simulink model "VCU_CS75_12_16_Test"  (R2014a)
settings: Solver=FixedStepDiscrete  StartTime=0.0  StopTime=25  FixedStep=0.0005  RelTol=1e-3
undefined symbols (not defined in the file): ecucoder_acal, I_SW01_L, LaterlAngleCommand, LDW, RemoteAcclPosition
libraries: simulink x913, ec5744lib x39
(part 1 of 30)
settings Model: Creator=pc  LastModifiedBy=ZJK
settings OptimizationCC: InlineParams=on  InlineInvariantSignals=on  ExpressionFolding=off  RollThreshold=9  StateBitsets=on  DataBitsets=on  UseTempVars=on  ZeroExternalMemoryAtStartup=off  ZeroInternalMemoryAtStartup=off  EfficientFloat2IntCast=on  OptimizeModelRefInitCode=on  LifeSpan=1
settings DebuggingCC: InheritedTsInSrcMsg=none  MultiTaskDSMMsg=none
settings HardwareCC: ProdLargestAtomicInteger=Long  ProdLargestAtomicFloat=Double  ProdIntDivRoundTo=Zero  ProdEndianess=BigEndian  ProdHWDeviceType=Freescale MPC5500
settings RTWCC: SystemTargetFile=ec5744.tlc  MakeCommand=make_rtw optimized_fixed_point=1  GenerateMakefile=off  TemplateMakefile=ec5744_lcc.tmf  PostCodeGenCommand=ec5744_pst_s2(buildInfo)  Description=Target for EC5744  GenerateReport=on  ProcessScript=ec5744_make_rtw_hook  IncludeHyperlinkInReport=on  LaunchReport=on
settings CodeAppCC: IgnoreCustomStorageClasses=off
settings STFCustomTargetCC: ModelReferenceCompliant=off  ConcurrentExecutionCompliant=off  IncludeMdlTerminateFcn=off  GeneratePreprocessorConditionals=Use local settings  CombineOutputUpdateFcns=on  SuppressErrorStatus=on  ERTCustomFileBanners=on  SupportContinuousTime=off  SupportNonInlinedSFcns=off  MATLABClassNameForMDSCustomization=Simulink.SoftwareTarget.ERTCustomization  GRTInterface=off  SystemTargetFile=ec5744.tlc
settings ERTTargetCC: GenerateSampleERTMain=off  ModelReferenceCompliant=off  IncludeMdlTerminateFcn=off  SuppressErrorStatus=on  GenerateASAP2=on  ERTSrcFileBannerTemplate=ec5744_code_template.cgt  ERTHdrFileBannerTemplate=ec5744_code_template.cgt  ERTDataSrcFileTemplate=ec5744_code_template.cgt  ERTDataHdrFileTemplate=ec5744_code_template.cgt  ERTCustomFileTemplate=ec5744_file_process.tlc

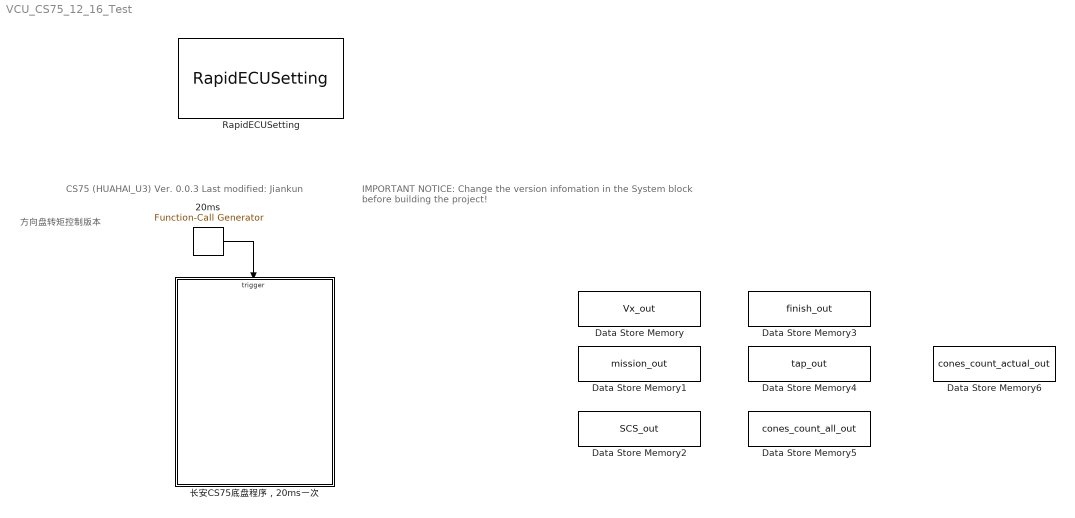
== system VCU_CS75_12_16_Test ==
  note: 方向盘转矩控制版本
  note: CS75 (HUAHAI_U3)
      | Ver. 0.0.3
      | Last modified: Jiankun
  note: IMPORTANT NOTICE:
      | Change the version infomation in the System block
      | before building the project!
  20ms : simulink/Ports & Subsystems/Function-Call Generator  sample_time=0.02  numberOfIterations=1
  Data Store Memory : DataStoreMemory  DataStoreName=Vx_out  ReadBeforeWriteMsg=warning  WriteAfterWriteMsg=warning  WriteAfterReadMsg=warning
  Data Store Memory1 : DataStoreMemory  DataStoreName=mission_out  ReadBeforeWriteMsg=warning  WriteAfterWriteMsg=warning  WriteAfterReadMsg=warning
  Data Store Memory2 : DataStoreMemory  DataStoreName=SCS_out  ReadBeforeWriteMsg=warning  WriteAfterWriteMsg=warning  WriteAfterReadMsg=warning
  Data Store Memory3 : DataStoreMemory  DataStoreName=finish_out  ReadBeforeWriteMsg=warning  WriteAfterWriteMsg=warning  WriteAfterReadMsg=warning
  Data Store Memory4 : DataStoreMemory  DataStoreName=tap_out  ReadBeforeWriteMsg=warning  WriteAfterWriteMsg=warning  WriteAfterReadMsg=warning
  Data Store Memory5 : DataStoreMemory  DataStoreName=cones_count_all_out  ReadBeforeWriteMsg=warning  WriteAfterWriteMsg=warning  WriteAfterReadMsg=warning
  Data Store Memory6 : DataStoreMemory  DataStoreName=cones_count_actual_out  ReadBeforeWriteMsg=warning  WriteAfterWriteMsg=warning  WriteAfterReadMsg=warning
  RapidECUSetting : ec5744lib/RapidECU_U3/RapidECUSetting
      link override CAN: apdf=4  bpdf=4  cpdf=4  acmt=Extended(29-bit ID)
      link override LIN: abrt=19200
  长安CS75底盘程序，20ms一次 : Subsystem
  wires:
  20ms/1 -> 长安CS75底盘程序，20ms一次/Trigger

== system VCU_CS75_12_16_Test/长安CS75底盘程序，20ms一次 ==
  Trigger : TriggerPort  TriggerType=function-call  PortDimensions=1
  APP : Subsystem  TreatAsAtomicUnit=on
  Input : Subsystem  TreatAsAtomicUnit=on
  Output : Subsystem
  wires:
  Input/1(IO_Input) -> APP/1(APP_Input)
  APP/1(APP_Output) -> Output/1(IO_Output)

== system VCU_CS75_12_16_Test/长安CS75底盘程序，20ms一次/APP ==
  note: 完全调试完需要修改一下，目前这个模块无用
  note: APP Module
      | Ver. 0.0.2
      | Last modified: ZJK 2020-10-09
  APP_Input : Inport
  Bus Creator1 : BusCreator
  Controller : Subsystem
  Monitor : Subsystem
  System_State_Manager : Subsystem
  APP_Output : Outport
  wires:
  Bus Creator1/1 -> APP_Output/1
  System_State_Manager/1(System_State) -> Bus Creator1/2, Controller/3(System_State)  "System_State"
  Monitor/1(System_Status) -> Bus Creator1/3, System_State_Manager/1(System_Status), Controller/2(System_Status)  "System_Status"
  Controller/1(Control_Output) -> Bus Creator1/1  "Control_Output"
  APP_Input/1 -> Controller/1(APP_Input), Bus Creator1/4, Monitor/1(APP_Input)  "APP_Input"

== system VCU_CS75_12_16_Test/长安CS75底盘程序，20ms一次/Input ==
  note: 程序版本-------方向盘转矩控制版本
  note: 接收底层发来的Messages
  note: 接收服务器Messages
  note: 低有效开关量6，用作横向自动驾驶开关
  note: Module
      | Ver. 0.0.1
      | Last modified by ZJK
  ADC_Input : Subsystem
  Bus Creator : BusCreator
  CAN0_Rx : Subsystem
  CAN1_Rx : Subsystem
  DBC转化的messages（存底） : Subsystem  Commented=on
  System : Subsystem  TreatAsAtomicUnit=on
  IO_Input : Outport
  wires:
  CAN0_Rx/1(CAN0_Data_Rx) -> Bus Creator/1  "CAN0_Data_Rx"
  CAN1_Rx/1(CAN1_Data_Rx) -> Bus Creator/2  "CAN1_Data_Rx"
  System/1(System_Output) -> Bus Creator/3  "System_Output"
  ADC_Input/1(ADC_Input) -> Bus Creator/4  "ADC_Input"
  Bus Creator/1 -> IO_Input/1

== system VCU_CS75_12_16_Test/长安CS75底盘程序，20ms一次/Output ==
  IO_Output : Inport
  CAN0_Tx : Subsystem
  CAN1_Tx : Subsystem
  Subsystem : Subsystem  Commented=on
  wires:
  IO_Output/1 -> CAN0_Tx/1(APP_Out), CAN1_Tx/1(APP_Out)

== system VCU_CS75_12_16_Test/长安CS75底盘程序，20ms一次/APP/Controller ==
  note: 方向盘震动控制，在退出和进入自动驾驶启用，目前未启用
  APP_Input : Inport
  System_Status : Inport  Port=2
  System_State : Inport  Port=3
  Accesories : Subsystem  TreatAsAtomicUnit=on
  Bus Creator : BusCreator  Inputs=5
  Bus Creator2 : BusCreator
  Bus Selector : BusSelector  OutputSignals=CAN0_Data_Rx,CAN1_Data_Rx,ADC_Input
  General : Subsystem  Commented=on  TreatAsAtomicUnit=on
  Lateral : Subsystem  TreatAsAtomicUnit=on
  Longitudinal : Subsystem  TreatAsAtomicUnit=on
  Control_Output : Outport
  wires:
  Bus Creator/1 -> General/1(Control_Input), Longitudinal/1(Control_Input), Accesories/1(Control_Input), Lateral/1(Control_Input)  "Control_Input"
  Bus Selector/1 -> Bus Creator/1  "<CAN0_Data_Rx>"
  APP_Input/1 -> Bus Selector/1
  Bus Selector/2 -> Bus Creator/2  "<CAN1_Data_Rx>"
  Accesories/1(Accesories_Output) -> Bus Creator2/4  "Accesories_Output"
  Lateral/1(Lateral_Output) -> Bus Creator2/3  "Lateral_Output"
  General/1(General_Output) -> Bus Creator2/1  "General_Output"
  Longitudinal/1(Longitudinal_Output) -> Bus Creator2/2  "Longitudinal_Output"
  Bus Creator2/1 -> Control_Output/1  "Control_Output"
  System_Status/1 -> Bus Creator/4  "System_Status"
  Bus Selector/3 -> Bus Creator/3  "<ADC_Input>"
  System_State/1 -> Bus Creator/5  "System_State"

== system VCU_CS75_12_16_Test/长安CS75底盘程序，20ms一次/APP/Monitor ==
  note: 网关发出EPS\ESP通讯或功能故障
  note: 人工接管状态（只要是制动踏板踩下，就认为驾驶员在控车）
  note: 服务器的通信状态/服务器下发的Ready信号
  note: 底层自己装的一个Switch，低有效
      | 可能用于判定进入自动驾驶的一个信号
  APP_Input : Inport
  Bus Creator : BusCreator
  Server_Status : Subsystem
  Switches_Status : Subsystem
  Vehicle_Status : Subsystem
  Vehicle_Takeover_Status : Subsystem
  System_Status : Outport
  wires:
  Bus Creator/1 -> System_Status/1
  APP_Input/1 -> [APP_Input]
  [APP_Input] -> Vehicle_Status/1(APP_Input)
  [APP_Input] -> Switches_Status/1(APP_Input)
  [APP_Input] -> Server_Status/1(APP_Input)
  [APP_Input] -> Vehicle_Takeover_Status/1(APP_Input)
  Vehicle_Status/1(Vehicle_Status) -> Bus Creator/1  "VehicleStatus"
  Vehicle_Takeover_Status/1(Takeover_Status) -> Bus Creator/2  "TakeOver1"
  Server_Status/1(Server_Status) -> Bus Creator/3  "ServerStatus"
  Switches_Status/1(Switches_Status) -> Bus Creator/4  "Switch_Status"

== system VCU_CS75_12_16_Test/长安CS75底盘程序，20ms一次/APP/System_State_Manager ==
  note: 暂时不考虑横向自动驾驶，目的是调试横向PID
  note: 0：人工驾驶；
      | 1：纵向自动驾驶；
      | 2：人工接管；
      | 3：底盘通信故障/功能故障；需要人工接管；
  System_Status : Inport
  Bus Selector : BusSelector  OutputSignals=VehicleStatus.VehicleFaultStatus,VehicleStatus.VehicleCommunicationStatus,VehicleStatus.EPS_AvailabilityStatus,TakeOver1,ServerStatus.Server_CommunicationStatus,ServerStatus.AutoDrivingReady,Switch_Status.P6_Value
  Chart : Stateflow chart  TreatAsAtomicUnit=on
  System_State : Outport
  wires:
  System_Status/1 -> Bus Selector/1
  Bus Selector/1 -> Chart/1(VehicleFaultStatus)  "<VehicleFaultStatus>"
  Bus Selector/2 -> Chart/2(VehicleComminicationStatus)  "<VehicleCommunicationStatus>"
  Bus Selector/4 -> Chart/4(TakeoverStatus)  "<TakeOver1>"
  Bus Selector/5 -> Chart/5(Server_CommunicationStatus)  "<Server_CommunicationStatus>"
  Bus Selector/6 -> Chart/6(AutoDrivingReady)  "<AutoDrivingReady>"
  Chart/1(System_State) -> System_State/1  "System_State"
  Bus Selector/7 -> Chart/7(Switch_P6)  "<P6_Value>"
  Bus Selector/3 -> Chart/3(EPS_AvailabilityStatus)  "<EPS_AvailabilityStatus>"

== system VCU_CS75_12_16_Test/长安CS75底盘程序，20ms一次/Input/ADC_Input ==
  Bus Creator2 : BusCreator  Inputs=1
  Data Type Conversion : DataTypeConversion  OutDataTypeStr=double
  MATLAB Function : MATLAB Function  TreatAsAtomicUnit=on
  SwitchInput : ec5744lib/RapidECU_U3/01BasicInput/SwitchInput  channel=6:I_SW01_L  sampletime=-1
  ADC_Input : Outport
  wires:
  SwitchInput/1 -> Data Type Conversion/1  "P6_Value"
  Bus Creator2/1 -> ADC_Input/1  "ADC_Input"
  Data Type Conversion/1 -> MATLAB Function/1(u)  "P6_Value"
  MATLAB Function/1(y) -> Bus Creator2/1  "P6_Value"

== system VCU_CS75_12_16_Test/长安CS75底盘程序，20ms一次/Input/CAN0_Rx ==
  note: BSW CAN 1 Receive
      | Communication to the vehicle
      | Ver. 1.0
      | 2020/11/14
  Bus Creator : BusCreator  Commented=on  Inputs=5
  Bus Creator2 : BusCreator  Inputs=1
  Constant : Constant  Commented=on  Value=0  SampleTime=-1
  Constant1 : Constant  Commented=on  Value=0  SampleTime=-1
  Constant2 : Constant  Commented=on  Value=0  SampleTime=-1
  ECCalVar1 : Constant  Commented=on  InitFcn=ecucoder_acal;  Value=RemoteAcclPosition  OutDataTypeStr=Inherit: Inherit via back propagation  SampleTime=-1
  ECCalVar2 : Constant  Commented=on  InitFcn=ecucoder_acal;  Value=LaterlAngleCommand  OutDataTypeStr=Inherit: Inherit via back propagation  SampleTime=-1
  a1_211 : Subsystem
  CAN0_Data_Rx : Outport
  wires:
  [A1_211] -> Bus Creator2/1  "A1_Data"
  Bus Creator2/1 -> CAN0_Data_Rx/1  "CAN0_Data_Rx"
  Bus Creator/1 -> ?
  Constant2/1 -> Bus Creator/1  "AutoDrivingReady"
  ECCalVar1/1 -> Bus Creator/2  "RemoteAcclPosition"
  ECCalVar2/1 -> Bus Creator/3  "LaterlAngleCommand"
  Constant/1 -> Bus Creator/4  "A1_Message_Counter"
  Constant1/1 -> Bus Creator/5  "A1_Checksum"
  a1_211/1(A1_211) -> [A1_211]

== system VCU_CS75_12_16_Test/长安CS75底盘程序，20ms一次/Input/CAN1_Rx ==
  BCM_288 : Subsystem
  BCM_328 : Subsystem
  BCM_348 : Subsystem
  BCM_3DF : Subsystem
  Bus Creator2 : BusCreator  Inputs=27
  EMS_205 : Subsystem
  EMS_255 : Subsystem
  EMS_265 : Subsystem
  EMS_276 : Subsystem
  EPB_256 : Subsystem
  EPS_20A : Subsystem
  EPS_21A : Subsystem
  ESP_277 : Subsystem
  ESP_280 : Subsystem
  ESP_281 : Subsystem
  ESP_287 : Subsystem
  GW_20B : Subsystem
  GW_308 : Subsystem
  GW_332 : Subsystem
  GW_376 : Subsystem
  GW_3A2 : Subsystem
  GW_567 : Subsystem
  HU_GPS_500 : Subsystem
  LAS_36E : Subsystem
  SAS_108 : Subsystem
  SCM_3B8 : Subsystem
  SRS_005 : Subsystem
  TCU_286 : Subsystem
  CAN1_Data_Rx : Outport
  wires:
  Bus Creator2/1 -> CAN1_Data_Rx/1  "CAN1_Data_Rx"
  [SAS_108] -> Bus Creator2/11  "SAS_108_Data"
  [BCM_328] -> Bus Creator2/16  "BCM_328_Data"
  [SCM_3B8] -> Bus Creator2/12  "SCM_3B8_Data"
  [GW_308] -> Bus Creator2/21  "GW_308_Data"
  [EMS_265] -> Bus Creator2/3  "EMS_265_Data"
  [ESP_287] -> Bus Creator2/10  "ESP_287_Data"
  [EPS_21A] -> Bus Creator2/6  "EPS_21A_Data"
  [ESP_277] -> Bus Creator2/7  "ESP_277_Data"
  [BCM_3DF] -> Bus Creator2/18  "BCM_3DF_Data"
  [ESP_281] -> Bus Creator2/9  "ESP_281_Data"
  [GW_332] -> Bus Creator2/20  "GW_332_Data"
  [ESP_280] -> Bus Creator2/8  "ESP_280_Data"
  [GW_20B] -> Bus Creator2/19  "GW_20B_Data"
  [BCM_348] -> Bus Creator2/17  "BCM_348_Data"
  [GW_376] -> Bus Creator2/22  "GW_376_Data"
  [SRS_005] -> Bus Creator2/13  "SRS_005_Data"
  [BCM_288] -> Bus Creator2/15  "BCM_288_Data"
  [TCU_286] -> Bus Creator2/14  "TCU_286_Data"
  [EPS_20A] -> Bus Creator2/5  "EPS_20A_Data"
  [EPB_256] -> Bus Creator2/4  "EPB_256_Data"
  [GW_3A2] -> Bus Creator2/23  "GW_3A2_Data"
  [GW_567] -> Bus Creator2/24  "GW_567_Data"
  [HU_GPS_500] -> Bus Creator2/25  "HU_GPS_500_Data"
  [LAS_36E] -> Bus Creator2/26  "LAS_36E_Data"
  [EMS_276] -> Bus Creator2/27  "EMS_276_Data"
  [EMS_205] -> Bus Creator2/1  "EMS_205_Data"
  [EMS_255] -> Bus Creator2/2  "EMS_255_Data"
  EMS_255/1(EMS_255) -> [EMS_255]
  EMS_265/1(EMS_265) -> [EMS_265]
  EMS_276/1(EMS_276) -> [EMS_276]
  EPB_256/1(EPB_256) -> [EPB_256]
  EMS_205/1(EMS_205) -> [EMS_205]
  EPS_20A/1(EPS_20A) -> [EPS_20A]
  EPS_21A/1(EPS_21A) -> [EPS_21A]
  ESP_277/1(ESP_277) -> [ESP_277]
  ESP_280/1(ESP_280) -> [ESP_280]
  ESP_281/1(ESP_281) -> [ESP_281]
  ESP_287/1(ESP_287) -> [ESP_287]
  SAS_108/1(SAS_108) -> [SAS_108]
  SCM_3B8/1(SCM_3B8) -> [SCM_3B8]
  SRS_005/1(SRS_005) -> [SRS_005]
  TCU_286/1(TCU_286) -> [TCU_286]
  BCM_288/1(BCM_288) -> [BCM_288]
  BCM_328/1(BCM_328) -> [BCM_328]
  BCM_348/1(BCM_348) -> [BCM_348]
  BCM_3DF/1(BCM_3DF) -> [BCM_3DF]
  GW_20B/1(GW_20B) -> [GW_20B]
  GW_332/1(GW_332) -> [GW_332]
  GW_308/1(GW_308) -> [GW_308]
  GW_376/1(GW_376) -> [GW_376]
  GW_3A2/1(GW_3A2) -> [GW_3A2]
  GW_567/1(GW_567) -> [GW_567]
  HU_GPS_500/1(HU_GPS_500) -> [HU_GPS_500]
  LAS_36E/1(LAS_36E) -> [LAS_36E]

== system VCU_CS75_12_16_Test/长安CS75底盘程序，20ms一次/Input/DBC转化的messages（存底） ==
  ReceiveMessages : Subsystem
  ReceiveMessages1 : Subsystem
  ReceiveMessages10 : Subsystem
  ReceiveMessages11 : Subsystem
  ReceiveMessages12 : Subsystem
  ReceiveMessages13 : Subsystem
  ReceiveMessages14 : Subsystem
  ReceiveMessages15 : Subsystem
  ReceiveMessages16 : Subsystem
  ReceiveMessages17 : Subsystem
  ReceiveMessages18 : Subsystem
  ReceiveMessages19 : Subsystem
  ReceiveMessages2 : Subsystem
  ReceiveMessages20 : Subsystem
  ReceiveMessages21 : Subsystem
  ReceiveMessages22 : Subsystem
  ReceiveMessages23 : Subsystem
  ReceiveMessages24 : Subsystem
  ReceiveMessages25 : Subsystem
  ReceiveMessages26 : Subsystem
  ReceiveMessages27 : Subsystem
  ReceiveMessages28 : Subsystem
  ReceiveMessages3 : Subsystem
  ReceiveMessages4 : Subsystem
  ReceiveMessages5 : Subsystem
  ReceiveMessages6 : Subsystem
  ReceiveMessages7 : Subsystem
  ReceiveMessages8 : Subsystem
  ReceiveMessages9 : Subsystem

== system VCU_CS75_12_16_Test/长安CS75底盘程序，20ms一次/Input/System ==
  Bus Creator : BusCreator  Inputs=1
  Bus Creator1 : BusCreator  Inputs=3
  Version_Major : Constant  Value=0  SampleTime=-1  LockScale=on
  Version_Minor : Constant  Value=0  SampleTime=-1
  Version_Patch : Constant  Value=2  SampleTime=-1
  System_Output : Outport
  wires:
  Bus Creator/1 -> System_Output/1  "System"
  Version_Minor/1 -> Bus Creator1/2  "Version_Minor"
  Version_Major/1 -> Bus Creator1/1  "Version_Major"
  Bus Creator1/1 -> Bus Creator/1  "Version"
  Version_Patch/1 -> Bus Creator1/3  "Version_Patch"

== system VCU_CS75_12_16_Test/长安CS75底盘程序，20ms一次/Output/CAN0_Tx ==
  note: BSW CAN0 Transmit
      | Communication to the Computer
      | Ver. 1.0
      | Last modified: ZJK 2020-10-05
  APP_Out : Inport
  From{,1..3} (4 alike) : From  Commented=on  GotoTag=APP_Signals
  to511 : Subsystem
  to6001 : Subsystem  Commented=on
  to6002 : Subsystem  Commented=on
  to6003 : Subsystem  Commented=on
  to6004 : Subsystem  Commented=on
  to601 : Subsystem
  wires:
  From/1 -> to6001/1(APP_Signals)
  APP_Out/1 -> [APP_Signals]
  From1/1 -> to6002/1(APP_Signals)
  From2/1 -> to6003/1(APP_Signals)
  From3/1 -> to6004/1(APP_Signals)
  [APP_Signals] -> to511/1(APP_Signals)
  [APP_Signals] -> to601/1(APP_Signals)

== system VCU_CS75_12_16_Test/长安CS75底盘程序，20ms一次/Output/CAN1_Tx ==
  note: BSW CAN 1 Transmit
      | Communication to the vehicle
      | Ver. 1.0
      | Last modified: ZJK 2020-
  APP_Out : Inport
  Bus Selector : BusSelector  Commented=on  OutputSignals=System_Status.Switch_Status.P6_Value
  From4 : From  Commented=on  GotoTag=APP_Signals
  Switch Case : SwitchCase  Commented=on  CaseConditions={0,1}  ShowDefaultCase=off
  Terminator : Terminator  Commented=on
  to28D : Subsystem
  to2E4 : Subsystem
  to2E5 : Subsystem
  wires:
  APP_Out/1 -> [APP_Signals]
  [APP_Signals] -> to2E4/1(APP_Signals)
  [APP_Signals] -> to2E5/1(APP_Signals)
  Switch Case/2 -> ?
  [APP_Signals] -> to28D/1(APP_Signals)
  From4/1 -> Bus Selector/1
  Bus Selector/1 -> Switch Case/1  "<P6_Value>"
  Switch Case/1 -> Terminator/1

== system VCU_CS75_12_16_Test/长安CS75底盘程序，20ms一次/Output/Subsystem ==
  28A : Subsystem
  28D : Subsystem
  2E4 : Subsystem
  2E5 : Subsystem
  TransmitMessages1 : Subsystem
  TransmitMessages10 : Subsystem
  TransmitMessages11 : Subsystem
  TransmitMessages13 : Subsystem
  TransmitMessages14 : Subsystem
  TransmitMessages2 : Subsystem
  TransmitMessages3 : Subsystem
  TransmitMessages4 : Subsystem
  TransmitMessages5 : Subsystem
  TransmitMessages7 : Subsystem
  TransmitMessages8 : Subsystem

== system VCU_CS75_12_16_Test/长安CS75底盘程序，20ms一次/APP/Controller/Accesories ==
  note: ID:28D
  note: 这里只有一个附加功能，方向盘震动；
      | 自己可以添加其他功能
  Control_Input : Inport
  Bus Creator : BusCreator  Inputs=2
  Bus Selector : BusSelector  OutputSignals=System_State
  ECCalVar : Constant  InitFcn=ecucoder_acal;  Value=LDW  OutDataTypeStr=Inherit: Inherit via back propagation  SampleTime=-1
  MATLAB Function : MATLAB Function  TreatAsAtomicUnit=on
  MATLAB Function1 : MATLAB Function  TreatAsAtomicUnit=on
  MATLAB Function2 : MATLAB Function  TreatAsAtomicUnit=on
  Memory2 : Memory  InheritSampleTime=on
  Accesories_Output : Outport
  wires:
  Control_Input/1 -> Bus Selector/1
  Bus Creator/1 -> Accesories_Output/1
  MATLAB Function/1(y1) -> Bus Creator/1  "LAS_LDWVibrationWarning"
  MATLAB Function/2(y2) -> Bus Creator/2  "LAS_LDWStatus"
  Memory2/1 -> MATLAB Function1/2(u2)
  Bus Selector/1 -> MATLAB Function2/1(u)  "<System_State>"
  MATLAB Function2/1(y) -> MATLAB Function1/1(u1), Memory2/1
  ECCalVar/1 -> MATLAB Function/1(u)

== system VCU_CS75_12_16_Test/长安CS75底盘程序，20ms一次/APP/Controller/General ==
  Control_Input : Inport
  Bus Creator : BusCreator  Inputs=1
  Bus Selector : BusSelector  OutputSignals=System_State
  MATLAB Function : MATLAB Function  TreatAsAtomicUnit=on
  General_Output : Outport
  wires:
  Bus Creator/1 -> General_Output/1
  MATLAB Function/1(y) -> Bus Creator/1  "ControlMode"
  Bus Selector/1 -> MATLAB Function/1(u)  "<System_State>"
  Control_Input/1 -> Bus Selector/1

== system VCU_CS75_12_16_Test/长安CS75底盘程序，20ms一次/APP/Controller/Lateral ==
  note: 查表
  note: 方向盘转角
  note: 轮胎转角
  note: 进入PID的信号
  note: 转矩输出
  note: 方向盘实际转角
  note: 目标控制转角
  note: 积分限幅
  note: 反馈的方向盘转角
  note: 转矩限幅
  note: 横向自动驾驶开关
  note: 转矩控制转向
  note: 位置式PID output = P*Error + I*ErrorSum + D*(Error - ErrorPre)
  note: 斜率控制，这里20才能让EPS不报警
  Control_Input : Inport
  1-D Lookup Table : Lookup_n-D  NumberOfTableDimensions=1  BreakpointsForDimension1=[-100 100]  Table=[-500 500]  InternalRulePriority=Speed  RndMeth=Simplest  InputSameDT=on
  Bus Creator1 : BusCreator  Inputs=6
  Bus Selector : BusSelector  OutputSignals=System_State,CAN0_Data_Rx.A1_Data.LaterlAngleCommand,System_Status.Switch_Status.P6_Value,CAN1_Data_Rx.TCU_286_Data.TCU_ActualGear,CAN1_Data_Rx.SAS_108_Data.SAS_SteeringAngle
  Constant : Constant  Value=0  SampleTime=-1
  Constant1 : Constant  SampleTime=-1
  Constant2 : Constant  Value=4  SampleTime=-1
  Constant3 : Constant  Value=0.2  SampleTime=-1
  Constant4 : Constant  Value=0  SampleTime=-1
  Constant5 : Constant  Value=1500  SampleTime=-1
  Constant6 : Constant  Value=3  SampleTime=-1
  Constant7 : Constant  Value=20  SampleTime=-1
  Data Type Conversion{1..4} (4 alike) : DataTypeConversion
  Gain1 : Gain  Gain=0.01
  MATLAB Function : MATLAB Function  TreatAsAtomicUnit=on
  MATLAB Function1 : MATLAB Function  TreatAsAtomicUnit=on
  MATLAB Function2 : MATLAB Function  TreatAsAtomicUnit=on
  MATLAB Function3 : MATLAB Function  TreatAsAtomicUnit=on
  MATLAB Function4 : MATLAB Function  TreatAsAtomicUnit=on
  MATLAB Function7 : MATLAB Function  TreatAsAtomicUnit=on
  Memory{1..4} (4 alike) : Memory  InheritSampleTime=on
  Switch : Switch  Criteria=u2 > Threshold
  Terminator : Terminator
  Lateral_Output : Outport
  wires:
  Control_Input/1 -> Bus Selector/1
  Bus Creator1/1 -> Lateral_Output/1  "28D"
  Bus Selector/2 -> [LaterlTorqueCommand]  "<LaterlAngleCommand>"
  Memory2/1 -> MATLAB Function2/2(LastCounter)
  Bus Selector/1 -> [System_State], MATLAB Function7/1(u)  "<System_State>"
  MATLAB Function7/1(y) -> [AutoDrivingMode]
  Bus Selector/3 -> [P6_Vaule]  "<P6_Value>"
  MATLAB Function3/1(LAS_Status) -> Bus Creator1/2  "LAS_LKSStatus"
  Bus Selector/4 -> [TCU_ActualGear]  "<TCU_ActualGear>"
  MATLAB Function4/1(y) -> Bus Creator1/1  "LAS_SteeringTorque"
  [System_State] -> MATLAB Function3/2(System_State)
  [P6_Vaule] -> MATLAB Function3/1(P6)
  Bus Selector/5 -> [SAS_SteeringAngle]  "<SAS_SteeringAngle>"
  [P6_Vaule] -> Switch/2
  Constant/1 -> Switch/3
  Switch/1 -> MATLAB Function4/1(T)
  Constant1/1 -> MATLAB Function2/1(Ready)
  MATLAB Function3/2(LateralTakeover) -> Terminator/1
  MATLAB Function2/1(RollingCounter) -> Memory2/1, Bus Creator1/3  "LAS_RollingCounter"
  [LaterlTorqueCommand] -> 1-D Lookup Table/1
  [SAS_SteeringAngle] -> MATLAB Function/2(SAS_SteeringAngle)
  [P6_Vaule] -> MATLAB Function/3(Ready)
  MATLAB Function/1(SteeringTorqueOut) -> MATLAB Function1/2(u1)  "PID_SteeringOut"
  MATLAB Function/3(ErrorSum) -> Data Type Conversion1/1  "ErrorSum"
  MATLAB Function/2(Error) -> Data Type Conversion2/1  "Error"
  Constant4/1 -> MATLAB Function/6(D)
  1-D Lookup Table/1 -> MATLAB Function/1(LaterlAngleCommand)  "mubiao_zhuanjiao"
  MATLAB Function1/1(y) -> Gain1/1, Memory4/1  "PID_SteeringTorque_out"
  Memory4/1 -> MATLAB Function1/3(u2)
  Gain1/1 -> Bus Creator1/4, Switch/1  "SteeringTorqueOut"
  Constant2/1 -> MATLAB Function/4(P)
  Constant5/1 -> MATLAB Function/7(ErrorSumMax)
  Constant7/1 -> MATLAB Function1/1(L1)
  Constant6/1 -> MATLAB Function4/2(Tmax)
  Memory1/1 -> Data Type Conversion3/1
  Memory3/1 -> Data Type Conversion4/1
  Data Type Conversion1/1 -> Memory1/1, Bus Creator1/5  "ErrorSum"
  Data Type Conversion2/1 -> Memory3/1, Bus Creator1/6  "Error"
  Data Type Conversion3/1 -> MATLAB Function/9(ErrorSumPre)
  Data Type Conversion4/1 -> MATLAB Function/8(ErrorPre)
  Constant3/1 -> MATLAB Function/5(I)

== system VCU_CS75_12_16_Test/长安CS75底盘程序，20ms一次/APP/Controller/Longitudinal ==
  note: 减速请求
  note: 起步泄压
  Control_Input : Inport
  Bus Creator : BusCreator  Inputs=6
  Bus Creator1 : BusCreator  Inputs=3
  Bus Creator2 : BusCreator  Inputs=2
  Bus Selector : BusSelector  OutputSignals=System_State,CAN0_Data_Rx.A1_Data.RemoteAcclPosition
  Constant : Constant  Value=3
  Constant1 : Constant  Value=0
  MATLAB Function : MATLAB Function  TreatAsAtomicUnit=on
  MATLAB Function1 : MATLAB Function  TreatAsAtomicUnit=on
  MATLAB Function2 : MATLAB Function  TreatAsAtomicUnit=on
  MATLAB Function3 : MATLAB Function  TreatAsAtomicUnit=on
  MATLAB Function4 : MATLAB Function  TreatAsAtomicUnit=on
  MATLAB Function5 : MATLAB Function  TreatAsAtomicUnit=on
  MATLAB Function6 : MATLAB Function  TreatAsAtomicUnit=on
  MATLAB Function7 : MATLAB Function  TreatAsAtomicUnit=on
  Memory1 : Memory  InheritSampleTime=on
  Memory2 : Memory  InheritSampleTime=on
  Saturation : Saturate  UpperLimit=0  LowerLimit=-5
  Saturation1 : Saturate  UpperLimit=10  LowerLimit=0
  Longitudinal_Output : Outport
  wires:
  Control_Input/1 -> Bus Selector/1
  MATLAB Function/1(y) -> Bus Creator/1  "ACC_CDDAxEnable"
  Constant1/1 -> Bus Creator/2  "ACC_DecToStop"
  MATLAB Function1/1(y) -> Bus Creator/3  "ACC_Driveoff_Request"
  Constant/1 -> Bus Creator/5  "ACC_Mode"
  MATLAB Function3/1(RollingCounter) -> Bus Creator/6, Memory1/1  "ACC_RollingCounter_id2E4"
  MATLAB Function5/1(y) -> Saturation1/1  "ACC_AccTorqueReq"
  MATLAB Function6/1(y) -> Bus Creator1/2  "ACC_TrqEnable"
  Bus Creator/1 -> Bus Creator2/1  "2E4"
  Bus Creator1/1 -> Bus Creator2/2  "2E5"
  Bus Creator2/1 -> Longitudinal_Output/1
  Bus Selector/2 -> [RemoteAcclPosition]  "<RemoteAcclPosition>"
  [RemoteAcclPosition] -> MATLAB Function/1(u), MATLAB Function1/1(u), MATLAB Function2/1(u1)
  MATLAB Function2/1(y) -> Saturation/1  "ACC_ACCTargetAcceleration"
  Memory1/1 -> MATLAB Function3/2(LastCounter)
  MATLAB Function4/1(RollingCounter) -> Memory2/1, Bus Creator1/3  "ACC_RollingCounter_id2E5"
  [AutoDrivingMode] -> MATLAB Function4/1(Ready), MATLAB Function5/1(u1), MATLAB Function3/1(Ready), MATLAB Function2/2(u2)
  Memory2/1 -> MATLAB Function4/2(LastCounter)
  [RemoteAcclPosition] -> MATLAB Function6/1(u), MATLAB Function5/2(u2)
  Bus Selector/1 -> MATLAB Function7/1(u)  "<System_State>"
  MATLAB Function7/1(y) -> [AutoDrivingMode]
  Saturation/1 -> Bus Creator/4  "ACC_ACCTargetAcceleration"
  Saturation1/1 -> Bus Creator1/1  "ACC_AccTorqueReq"

== system VCU_CS75_12_16_Test/长安CS75底盘程序，20ms一次/APP/Monitor/Server_Status ==
  APP_Input : Inport
  1s1 : Constant  Value=1000
  Bus Creator : BusCreator  Inputs=2
  Bus Selector : BusSelector  OutputSignals=CAN0_Data_Rx.A1_Data.A1_Message_Counter,CAN0_Data_Rx.A1_Data.AutoDrivingReady
  Constant : Constant  SampleTime=-1
  MATLAB Function1 : MATLAB Function  TreatAsAtomicUnit=on
  Memory1 : Memory  InheritSampleTime=on
  Memory2 : Memory  InheritSampleTime=on
  Terminator : Terminator
  Server_Status : Outport
  wires:
  APP_Input/1 -> Bus Selector/1
  Bus Selector/2 -> Bus Creator/2  "<AutoDrivingReady>"
  Bus Creator/1 -> Server_Status/1  "ServerStatus"
  1s1/1 -> MATLAB Function1/1(TimeThreshold)
  Bus Selector/1 -> MATLAB Function1/2(RollingCounter), Memory1/1  "<A1_Message_Counter>"
  MATLAB Function1/2(Counter) -> Memory2/1  "counter3"
  Memory2/1 -> MATLAB Function1/4(LastCounter)
  Constant/1 -> Bus Creator/1  "Server_CommunicationStatus"
  Memory1/1 -> MATLAB Function1/3(LastRollingCounter)  "A1counter"
  MATLAB Function1/1(EPS_CommunicationStatus) -> Terminator/1

== system VCU_CS75_12_16_Test/长安CS75底盘程序，20ms一次/APP/Monitor/Switches_Status ==
  APP_Input : Inport
  Bus Creator : BusCreator  Inputs=1
  Bus Selector : BusSelector  OutputSignals=ADC_Input.P6_Value
  Switches_Status : Outport
  wires:
  APP_Input/1 -> Bus Selector/1
  Bus Selector/1 -> Bus Creator/1  "<P6_Value>"
  Bus Creator/1 -> Switches_Status/1  "Switch_Status"

== system VCU_CS75_12_16_Test/长安CS75底盘程序，20ms一次/APP/Monitor/Vehicle_Status ==
  note: APA转角控制握手反馈
  APP_Input : Inport
  1s : Constant  Value=1000
  Bus Creator : BusCreator  Inputs=3
  Bus Selector : BusSelector  OutputSignals=CAN1_Data_Rx.EPS_20A_Data.EPS_EPSFailed,CAN1_Data_Rx.ESP_281_Data.ESP_ESPFailStatus,CAN1_Data_Rx.EMS_255_Data.EMS_RollingCounter_id255,CAN1_Data_Rx.EPS_21A_Data.EPS_AvailabilityStatus
  Data Type Conversion : DataTypeConversion
  MATLAB Function2 : MATLAB Function  TreatAsAtomicUnit=on
  MATLAB Function4 : MATLAB Function  TreatAsAtomicUnit=on
  Memory2 : Memory  InheritSampleTime=on
  Memory3 : Memory  InheritSampleTime=on
  Signal Conversion : SignalConversion
  Vehicle_Status : Outport
  wires:
  Bus Selector/1 -> MATLAB Function2/1(u1)  "<EPS_EPSFailed>"
  MATLAB Function4/1(EPS_CommunicationStatus) -> Bus Creator/2  "VehicleCommunicationStatus"
  1s/1 -> MATLAB Function4/1(TimeThreshold)
  Bus Creator/1 -> Vehicle_Status/1  "VehicleStatus"
  MATLAB Function2/1(y) -> Bus Creator/1  "VehicleFaultStatus"
  Bus Selector/3 -> MATLAB Function4/2(RollingCounter), Memory3/1  "<EMS_RollingCounter_id255>"
  Bus Selector/2 -> MATLAB Function2/2(u2)  "<ESP_ESPFailStatus>"
  Memory3/1 -> MATLAB Function4/3(LastRollingCounter)
  MATLAB Function4/2(Counter) -> Memory2/1  "counter1"
  Memory2/1 -> MATLAB Function4/4(LastCounter)
  APP_Input/1 -> Signal Conversion/1
  Signal Conversion/1 -> Bus Selector/1
  Bus Selector/4 -> Data Type Conversion/1  "<EPS_AvailabilityStatus>"
  Data Type Conversion/1 -> Bus Creator/3  "EPS_AvailabilityStatus"

== system VCU_CS75_12_16_Test/长安CS75底盘程序，20ms一次/APP/Monitor/Vehicle_Takeover_Status ==
  APP_Input : Inport
  AccelPedalTakeover : Constant  Value=0
  Bus Selector : BusSelector  OutputSignals=CAN1_Data_Rx.EMS_255_Data.EMS_BrakePedalStatus
  SteeringTakeover : Constant  Value=0
  Terminator : Terminator
  Terminator1 : Terminator
  Takeover_Status : Outport
  wires:
  APP_Input/1 -> Bus Selector/1
  AccelPedalTakeover/1 -> Terminator1/1
  SteeringTakeover/1 -> Terminator/1
  Bus Selector/1 -> Takeover_Status/1  "<EMS_BrakePedalStatus>"

== system VCU_CS75_12_16_Test/长安CS75底盘程序，20ms一次/Input/CAN0_Rx/a1_211 ==
  CANReceive : ec5744lib/RapidECU_U3/04CANCommunication/CANReceive  canmodule=0  canbuffer=0  canmessageid=hex2dec('211')  canmessagetype=Standard(11-bit ID)  datalength=8  sampletime=-1
  ReceiveMessages : Subsystem
  Terminator : Terminator
  Terminator1 : Terminator
  A1_211 : Outport
  wires:
  ReceiveMessages/1(A1_211) -> A1_211/1
  CANReceive/3 -> Terminator/1
  CANReceive/4 -> ReceiveMessages/2(In2)
  CANReceive/1 -> ReceiveMessages/Trigger
  CANReceive/2 -> ReceiveMessages/1(In1)
  CANReceive/5 -> Terminator1/1

== system VCU_CS75_12_16_Test/长安CS75底盘程序，20ms一次/Input/CAN1_Rx/BCM_288 ==
  CANReceive : ec5744lib/RapidECU_U3/04CANCommunication/CANReceive  canmodule=1  canbuffer=23  canmessageid=hex2dec('288')  canmessagetype=Standard(11-bit ID)  datalength=8  sampletime=-1
  ReceiveMessages : Subsystem
  Terminator : Terminator
  Terminator1 : Terminator
  BCM_288 : Outport
  wires:
  CANReceive/5 -> Terminator1/1
  CANReceive/2 -> ReceiveMessages/1(In1)
  CANReceive/1 -> ReceiveMessages/Trigger
  CANReceive/4 -> ReceiveMessages/2(In2)
  CANReceive/3 -> Terminator/1
  ReceiveMessages/1(BCM_288) -> BCM_288/1

== system VCU_CS75_12_16_Test/长安CS75底盘程序，20ms一次/Input/CAN1_Rx/BCM_328 ==
  CANReceive : ec5744lib/RapidECU_U3/04CANCommunication/CANReceive  canmodule=1  canbuffer=24  canmessageid=hex2dec('328')  canmessagetype=Standard(11-bit ID)  datalength=8  sampletime=-1
  ReceiveMessages : Subsystem
  Terminator : Terminator
  Terminator1 : Terminator
  BCM_328 : Outport
  wires:
  ReceiveMessages/1(BCM_328) -> BCM_328/1
  CANReceive/3 -> Terminator/1
  CANReceive/4 -> ReceiveMessages/2(In2)
  CANReceive/1 -> ReceiveMessages/Trigger
  CANReceive/2 -> ReceiveMessages/1(In1)
  CANReceive/5 -> Terminator1/1

== system VCU_CS75_12_16_Test/长安CS75底盘程序，20ms一次/Input/CAN1_Rx/BCM_348 ==
  CANReceive : ec5744lib/RapidECU_U3/04CANCommunication/CANReceive  canmodule=1  canbuffer=25  canmessageid=hex2dec('348')  canmessagetype=Standard(11-bit ID)  datalength=8  sampletime=-1
  ReceiveMessages : Subsystem
  Terminator : Terminator
  Terminator1 : Terminator
  BCM_348 : Outport
  wires:
  CANReceive/5 -> Terminator1/1
  CANReceive/2 -> ReceiveMessages/1(In1)
  CANReceive/1 -> ReceiveMessages/Trigger
  CANReceive/4 -> ReceiveMessages/2(In2)
  CANReceive/3 -> Terminator/1
  ReceiveMessages/1(BCM_348) -> BCM_348/1

== system VCU_CS75_12_16_Test/长安CS75底盘程序，20ms一次/Input/CAN1_Rx/BCM_3DF ==
  CANReceive : ec5744lib/RapidECU_U3/04CANCommunication/CANReceive  canmodule=1  canbuffer=26  canmessageid=hex2dec('3DF')  canmessagetype=Standard(11-bit ID)  datalength=8  sampletime=-1
  ReceiveMessages : Subsystem
  Terminator : Terminator
  Terminator1 : Terminator
  BCM_3DF : Outport
  wires:
  ReceiveMessages/1(BCM_3DF) -> BCM_3DF/1
  CANReceive/3 -> Terminator/1
  CANReceive/4 -> ReceiveMessages/2(In2)
  CANReceive/1 -> ReceiveMessages/Trigger
  CANReceive/2 -> ReceiveMessages/1(In1)
  CANReceive/5 -> Terminator1/1

== system VCU_CS75_12_16_Test/长安CS75底盘程序，20ms一次/Input/CAN1_Rx/EMS_205 ==
  CANReceive : ec5744lib/RapidECU_U3/04CANCommunication/CANReceive  canmodule=1  canbuffer=0  canmessageid=hex2dec('205')  canmessagetype=Standard(11-bit ID)  datalength=8  sampletime=-1
  ReceiveMessages : Subsystem
  Terminator : Terminator
  Terminator1 : Terminator
  EMS_205 : Outport
  wires:
  ReceiveMessages/1(EMS_205) -> EMS_205/1
  CANReceive/3 -> Terminator/1
  CANReceive/4 -> ReceiveMessages/2(In2)
  CANReceive/1 -> ReceiveMessages/Trigger
  CANReceive/2 -> ReceiveMessages/1(In1)
  CANReceive/5 -> Terminator1/1

== system VCU_CS75_12_16_Test/长安CS75底盘程序，20ms一次/Input/CAN1_Rx/EMS_255 ==
  CANReceive : ec5744lib/RapidECU_U3/04CANCommunication/CANReceive  canmodule=1  canbuffer=1  canmessageid=hex2dec('255')  canmessagetype=Standard(11-bit ID)  datalength=8  sampletime=-1
  ReceiveMessages : Subsystem
  Terminator : Terminator
  Terminator1 : Terminator
  EMS_255 : Outport
  wires:
  CANReceive/5 -> Terminator1/1
  CANReceive/2 -> ReceiveMessages/1(In1)
  CANReceive/1 -> ReceiveMessages/Trigger
  CANReceive/4 -> ReceiveMessages/2(In2)
  CANReceive/3 -> Terminator/1
  ReceiveMessages/1(EMS_255) -> EMS_255/1

== system VCU_CS75_12_16_Test/长安CS75底盘程序，20ms一次/Input/CAN1_Rx/EMS_265 ==
  CANReceive : ec5744lib/RapidECU_U3/04CANCommunication/CANReceive  canmodule=1  canbuffer=2  canmessageid=hex2dec('265')  canmessagetype=Standard(11-bit ID)  datalength=8  sampletime=-1
  ReceiveMessages : Subsystem
  Terminator : Terminator
  Terminator1 : Terminator
  EMS_265 : Outport
  wires:
  ReceiveMessages/1(EMS_265) -> EMS_265/1
  CANReceive/3 -> Terminator/1
  CANReceive/4 -> ReceiveMessages/2(In2)
  CANReceive/1 -> ReceiveMessages/Trigger
  CANReceive/2 -> ReceiveMessages/1(In1)
  CANReceive/5 -> Terminator1/1

== system VCU_CS75_12_16_Test/长安CS75底盘程序，20ms一次/Input/CAN1_Rx/EMS_276 ==
  CANReceive : ec5744lib/RapidECU_U3/04CANCommunication/CANReceive  canmodule=1  canbuffer=3  canmessageid=hex2dec('276')  canmessagetype=Standard(11-bit ID)  datalength=8  sampletime=-1
  ReceiveMessages : Subsystem
  Terminator : Terminator
  Terminator1 : Terminator
  EMS_276 : Outport
  wires:
  CANReceive/5 -> Terminator1/1
  CANReceive/2 -> ReceiveMessages/1(In1)
  CANReceive/1 -> ReceiveMessages/Trigger
  CANReceive/4 -> ReceiveMessages/2(In2)
  CANReceive/3 -> Terminator/1
  ReceiveMessages/1(EMS_276) -> EMS_276/1

== system VCU_CS75_12_16_Test/长安CS75底盘程序，20ms一次/Input/CAN1_Rx/EPB_256 ==
  CANReceive : ec5744lib/RapidECU_U3/04CANCommunication/CANReceive  canmodule=1  canbuffer=4  canmessageid=hex2dec('256')  canmessagetype=Standard(11-bit ID)  datalength=8  sampletime=-1
  ReceiveMessages : Subsystem
  Terminator : Terminator
  Terminator1 : Terminator
  EPB_256 : Outport
  wires:
  ReceiveMessages/1(EMS_256) -> EPB_256/1
  CANReceive/3 -> Terminator/1
  CANReceive/4 -> ReceiveMessages/2(In2)
  CANReceive/1 -> ReceiveMessages/Trigger
  CANReceive/2 -> ReceiveMessages/1(In1)
  CANReceive/5 -> Terminator1/1

== system VCU_CS75_12_16_Test/长安CS75底盘程序，20ms一次/Input/CAN1_Rx/EPS_20A ==
  CANReceive : ec5744lib/RapidECU_U3/04CANCommunication/CANReceive  canmodule=1  canbuffer=5  canmessageid=hex2dec('20A')  canmessagetype=Standard(11-bit ID)  datalength=8  sampletime=-1
  ReceiveMessages : Subsystem
  Terminator : Terminator
  Terminator1 : Terminator
  EPS_20A : Outport
  wires:
  CANReceive/5 -> Terminator1/1
  CANReceive/2 -> ReceiveMessages/1(In1)
  CANReceive/1 -> ReceiveMessages/Trigger
  CANReceive/4 -> ReceiveMessages/2(In2)
  CANReceive/3 -> Terminator/1
  ReceiveMessages/1(EPS_20A) -> EPS_20A/1

== system VCU_CS75_12_16_Test/长安CS75底盘程序，20ms一次/Input/CAN1_Rx/EPS_21A ==
  CANReceive : ec5744lib/RapidECU_U3/04CANCommunication/CANReceive  canmodule=1  canbuffer=6  canmessageid=hex2dec('21A')  canmessagetype=Standard(11-bit ID)  datalength=8  sampletime=-1
  ReceiveMessages : Subsystem
  Terminator : Terminator
  Terminator1 : Terminator
  EPS_21A : Outport
  wires:
  ReceiveMessages/1(EPS_21A) -> EPS_21A/1
  CANReceive/3 -> Terminator/1
  CANReceive/4 -> ReceiveMessages/2(In2)
  CANReceive/1 -> ReceiveMessages/Trigger
  CANReceive/2 -> ReceiveMessages/1(In1)
  CANReceive/5 -> Terminator1/1

== system VCU_CS75_12_16_Test/长安CS75底盘程序，20ms一次/Input/CAN1_Rx/ESP_277 ==
  CANReceive : ec5744lib/RapidECU_U3/04CANCommunication/CANReceive  canmodule=1  canbuffer=7  canmessageid=hex2dec('277')  canmessagetype=Standard(11-bit ID)  datalength=8  sampletime=-1
  ReceiveMessages : Subsystem
  Terminator : Terminator
  Terminator1 : Terminator
  ESP_277 : Outport
  wires:
  CANReceive/5 -> Terminator1/1
  CANReceive/2 -> ReceiveMessages/1(In1)
  CANReceive/1 -> ReceiveMessages/Trigger
  CANReceive/4 -> ReceiveMessages/2(In2)
  CANReceive/3 -> Terminator/1
  ReceiveMessages/1(ESP_277) -> ESP_277/1

== system VCU_CS75_12_16_Test/长安CS75底盘程序，20ms一次/Input/CAN1_Rx/ESP_280 ==
  CANReceive : ec5744lib/RapidECU_U3/04CANCommunication/CANReceive  canmodule=1  canbuffer=16  canmessageid=hex2dec('280')  canmessagetype=Standard(11-bit ID)  datalength=8  sampletime=-1
  ReceiveMessages : Subsystem
  Terminator : Terminator
  Terminator1 : Terminator
  ESP_280 : Outport
  wires:
  ReceiveMessages/1(ESP_280) -> ESP_280/1
  CANReceive/3 -> Terminator/1
  CANReceive/4 -> ReceiveMessages/2(In2)
  CANReceive/1 -> ReceiveMessages/Trigger
  CANReceive/2 -> ReceiveMessages/1(In1)
  CANReceive/5 -> Terminator1/1

== system VCU_CS75_12_16_Test/长安CS75底盘程序，20ms一次/Input/CAN1_Rx/ESP_281 ==
  CANReceive : ec5744lib/RapidECU_U3/04CANCommunication/CANReceive  canmodule=1  canbuffer=17  canmessageid=hex2dec('281')  canmessagetype=Standard(11-bit ID)  datalength=8  sampletime=-1
  ReceiveMessages : Subsystem
  Terminator : Terminator
  Terminator1 : Terminator
  ESP_281 : Outport
  wires:
  CANReceive/5 -> Terminator1/1
  CANReceive/2 -> ReceiveMessages/1(In1)
  CANReceive/1 -> ReceiveMessages/Trigger
  CANReceive/4 -> ReceiveMessages/2(In2)
  CANReceive/3 -> Terminator/1
  ReceiveMessages/1(ESP_281) -> ESP_281/1

== system VCU_CS75_12_16_Test/长安CS75底盘程序，20ms一次/Input/CAN1_Rx/ESP_287 ==
  CANReceive : ec5744lib/RapidECU_U3/04CANCommunication/CANReceive  canmodule=1  canbuffer=18  canmessageid=hex2dec('287')  canmessagetype=Standard(11-bit ID)  datalength=8  sampletime=-1
  ReceiveMessages : Subsystem
  Terminator : Terminator
  Terminator1 : Terminator
  ESP_287 : Outport
  wires:
  ReceiveMessages/1(ESP_287) -> ESP_287/1
  CANReceive/3 -> Terminator/1
  CANReceive/4 -> ReceiveMessages/2(In2)
  CANReceive/1 -> ReceiveMessages/Trigger
  CANReceive/2 -> ReceiveMessages/1(In1)
  CANReceive/5 -> Terminator1/1

== system VCU_CS75_12_16_Test/长安CS75底盘程序，20ms一次/Input/CAN1_Rx/GW_20B ==
  CANReceive : ec5744lib/RapidECU_U3/04CANCommunication/CANReceive  canmodule=1  canbuffer=27  canmessageid=hex2dec('20B')  canmessagetype=Standard(11-bit ID)  datalength=8  sampletime=-1
  ReceiveMessages : Subsystem
  Terminator : Terminator
  Terminator1 : Terminator
  GW_20B : Outport
  wires:
  CANReceive/5 -> Terminator1/1
  CANReceive/2 -> ReceiveMessages/1(In1)
  CANReceive/1 -> ReceiveMessages/Trigger
  CANReceive/4 -> ReceiveMessages/2(In2)
  CANReceive/3 -> Terminator/1
  ReceiveMessages/1(GW_20B) -> GW_20B/1

== system VCU_CS75_12_16_Test/长安CS75底盘程序，20ms一次/Input/CAN1_Rx/GW_308 ==
  CANReceive : ec5744lib/RapidECU_U3/04CANCommunication/CANReceive  canmodule=1  canbuffer=29  canmessageid=hex2dec('308')  canmessagetype=Standard(11-bit ID)  datalength=8  sampletime=-1
  ReceiveMessages : Subsystem
  Terminator : Terminator
  Terminator1 : Terminator
  GW_308 : Outport
  wires:
  CANReceive/5 -> Terminator1/1
  CANReceive/2 -> ReceiveMessages/1(In1)
  CANReceive/1 -> ReceiveMessages/Trigger
  CANReceive/4 -> ReceiveMessages/2(In2)
  CANReceive/3 -> Terminator/1
  ReceiveMessages/1(GW_308) -> GW_308/1

== system VCU_CS75_12_16_Test/长安CS75底盘程序，20ms一次/Input/CAN1_Rx/GW_332 ==
  CANReceive : ec5744lib/RapidECU_U3/04CANCommunication/CANReceive  canmodule=1  canbuffer=28  canmessageid=hex2dec('332')  canmessagetype=Standard(11-bit ID)  datalength=8  sampletime=-1
  ReceiveMessages : Subsystem
  Terminator : Terminator
  Terminator1 : Terminator
  GW_332 : Outport
  wires:
  ReceiveMessages/1(GW_332) -> GW_332/1
  CANReceive/3 -> Terminator/1
  CANReceive/4 -> ReceiveMessages/2(In2)
  CANReceive/1 -> ReceiveMessages/Trigger
  CANReceive/2 -> ReceiveMessages/1(In1)
  CANReceive/5 -> Terminator1/1

== system VCU_CS75_12_16_Test/长安CS75底盘程序，20ms一次/Input/CAN1_Rx/GW_376 ==
  CANReceive : ec5744lib/RapidECU_U3/04CANCommunication/CANReceive  canmodule=1  canbuffer=30  canmessageid=hex2dec('376')  canmessagetype=Standard(11-bit ID)  datalength=8  sampletime=-1
  ReceiveMessages : Subsystem
  Terminator : Terminator
  Terminator1 : Terminator
  GW_376 : Outport
  wires:
  ReceiveMessages/1(GW_376) -> GW_376/1
  CANReceive/3 -> Terminator/1
  CANReceive/4 -> ReceiveMessages/2(In2)
  CANReceive/1 -> ReceiveMessages/Trigger
  CANReceive/2 -> ReceiveMessages/1(In1)
  CANReceive/5 -> Terminator1/1

== system VCU_CS75_12_16_Test/长安CS75底盘程序，20ms一次/Input/CAN1_Rx/GW_3A2 ==
  CANReceive : ec5744lib/RapidECU_U3/04CANCommunication/CANReceive  canmodule=1  canbuffer=31  canmessageid=hex2dec('3A2')  canmessagetype=Standard(11-bit ID)  datalength=8  sampletime=-1
  ReceiveMessages : Subsystem
  Terminator : Terminator
  Terminator1 : Terminator
  GW_3A2 : Outport
  wires:
  CANReceive/5 -> Terminator1/1
  CANReceive/2 -> ReceiveMessages/1(In1)
  CANReceive/1 -> ReceiveMessages/Trigger
  CANReceive/4 -> ReceiveMessages/2(In2)
  CANReceive/3 -> Terminator/1
  ReceiveMessages/1(GW_3A2) -> GW_3A2/1

== system VCU_CS75_12_16_Test/长安CS75底盘程序，20ms一次/Input/CAN1_Rx/GW_567 ==
  CANReceive : ec5744lib/RapidECU_U3/04CANCommunication/CANReceive  canmodule=1  canbuffer=32  canmessageid=hex2dec('567')  canmessagetype=Standard(11-bit ID)  datalength=8  sampletime=-1
  ReceiveMessages : Subsystem
  Terminator : Terminator
  Terminator1 : Terminator
  GW_567 : Outport
  wires:
  ReceiveMessages/1(GW_567) -> GW_567/1
  CANReceive/3 -> Terminator/1
  CANReceive/4 -> ReceiveMessages/2(In2)
  CANReceive/1 -> ReceiveMessages/Trigger
  CANReceive/2 -> ReceiveMessages/1(In1)
  CANReceive/5 -> Terminator1/1

== system VCU_CS75_12_16_Test/长安CS75底盘程序，20ms一次/Input/CAN1_Rx/HU_GPS_500 ==
  CANReceive : ec5744lib/RapidECU_U3/04CANCommunication/CANReceive  canmodule=1  canbuffer=33  canmessageid=hex2dec('500')  canmessagetype=Standard(11-bit ID)  datalength=8  sampletime=-1
  ReceiveMessages : Subsystem
  Terminator : Terminator
  Terminator1 : Terminator
  HU_GPS_500 : Outport
  wires:
  CANReceive/5 -> Terminator1/1
  CANReceive/2 -> ReceiveMessages/1(In1)
  CANReceive/1 -> ReceiveMessages/Trigger
  CANReceive/4 -> ReceiveMessages/2(In2)
  CANReceive/3 -> Terminator/1
  ReceiveMessages/1(HU_GPS_500) -> HU_GPS_500/1

== system VCU_CS75_12_16_Test/长安CS75底盘程序，20ms一次/Input/CAN1_Rx/LAS_36E ==
  CANReceive : ec5744lib/RapidECU_U3/04CANCommunication/CANReceive  canmodule=1  canbuffer=36  canmessageid=hex2dec('36E')  canmessagetype=Standard(11-bit ID)  datalength=8  sampletime=-1
  ReceiveMessages : Subsystem
  Terminator : Terminator
  Terminator1 : Terminator
  LAS_36E : Outport
  wires:
  ReceiveMessages/1(LAS_36E) -> LAS_36E/1
  CANReceive/3 -> Terminator/1
  CANReceive/4 -> ReceiveMessages/2(In2)
  CANReceive/1 -> ReceiveMessages/Trigger
  CANReceive/2 -> ReceiveMessages/1(In1)
  CANReceive/5 -> Terminator1/1

== system VCU_CS75_12_16_Test/长安CS75底盘程序，20ms一次/Input/CAN1_Rx/SAS_108 ==
  CANReceive : ec5744lib/RapidECU_U3/04CANCommunication/CANReceive  canmodule=1  canbuffer=19  canmessageid=hex2dec('108')  canmessagetype=Standard(11-bit ID)  datalength=8  sampletime=-1
  ReceiveMessages : Subsystem
  Terminator : Terminator
  Terminator1 : Terminator
  SAS_108 : Outport
  wires:
  CANReceive/5 -> Terminator1/1
  CANReceive/2 -> ReceiveMessages/1(In1)
  CANReceive/1 -> ReceiveMessages/Trigger
  CANReceive/4 -> ReceiveMessages/2(In2)
  CANReceive/3 -> Terminator/1
  ReceiveMessages/1(SAS_108) -> SAS_108/1

== system VCU_CS75_12_16_Test/长安CS75底盘程序，20ms一次/Input/CAN1_Rx/SCM_3B8 ==
  CANReceive : ec5744lib/RapidECU_U3/04CANCommunication/CANReceive  canmodule=1  canbuffer=20  canmessageid=hex2dec('3B8')  canmessagetype=Standard(11-bit ID)  datalength=8  sampletime=-1
  ReceiveMessages : Subsystem
  Terminator : Terminator
  Terminator1 : Terminator
  SCM_3B8 : Outport
  wires:
  ReceiveMessages/1(SCM_3B8) -> SCM_3B8/1
  CANReceive/3 -> Terminator/1
  CANReceive/4 -> ReceiveMessages/2(In2)
  CANReceive/1 -> ReceiveMessages/Trigger
  CANReceive/2 -> ReceiveMessages/1(In1)
  CANReceive/5 -> Terminator1/1

== system VCU_CS75_12_16_Test/长安CS75底盘程序，20ms一次/Input/CAN1_Rx/SRS_005 ==
  CANReceive : ec5744lib/RapidECU_U3/04CANCommunication/CANReceive  canmodule=1  canbuffer=21  canmessageid=hex2dec('005')  canmessagetype=Standard(11-bit ID)  datalength=8  sampletime=-1
  ReceiveMessages : Subsystem
  Terminator : Terminator
  Terminator1 : Terminator
  SRS_005 : Outport
  wires:
  CANReceive/5 -> Terminator1/1
  CANReceive/2 -> ReceiveMessages/1(In1)
  CANReceive/1 -> ReceiveMessages/Trigger
  CANReceive/4 -> ReceiveMessages/2(In2)
  CANReceive/3 -> Terminator/1
  ReceiveMessages/1(SRS_005) -> SRS_005/1

== system VCU_CS75_12_16_Test/长安CS75底盘程序，20ms一次/Input/CAN1_Rx/TCU_286 ==
  CANReceive : ec5744lib/RapidECU_U3/04CANCommunication/CANReceive  canmodule=1  canbuffer=22  canmessageid=hex2dec('286')  canmessagetype=Standard(11-bit ID)  datalength=8  sampletime=-1
  ReceiveMessages : Subsystem
  Terminator : Terminator
  Terminator1 : Terminator
  TCU_286 : Outport
  wires:
  ReceiveMessages/1(TCU_286) -> TCU_286/1
  CANReceive/3 -> Terminator/1
  CANReceive/4 -> ReceiveMessages/2(In2)
  CANReceive/1 -> ReceiveMessages/Trigger
  CANReceive/2 -> ReceiveMessages/1(In1)
  CANReceive/5 -> Terminator1/1

== system VCU_CS75_12_16_Test/长安CS75底盘程序，20ms一次/Input/DBC转化的messages（存底）/ReceiveMessages ==
  EMS_205 : Subsystem
  EMS_205_GND : Ground
  EMS_CheckSum_205_Ter : Terminator
  EMS_ESPTorqReuestAvailability_Ter : Terminator
  EMS_FrictionalTorq_Ter : Terminator
  EMS_IndicatedDriverReqTorq_Ter : Terminator
  EMS_IndicatedRealEngTorq_Ter : Terminator
  EMS_RollingCounter_id205_Ter : Terminator
  EMS_TorqFailure_Ter : Terminator
  wires:
  EMS_205/1(EMS_ESPTorqReuestAvailability_Out) -> EMS_ESPTorqReuestAvailability_Ter/1
  EMS_205/2(EMS_TorqFailure_Out) -> EMS_TorqFailure_Ter/1
  EMS_205/3(EMS_IndicatedDriverReqTorq_Out) -> EMS_IndicatedDriverReqTorq_Ter/1
  EMS_205/4(EMS_FrictionalTorq_Out) -> EMS_FrictionalTorq_Ter/1
  EMS_205/5(EMS_IndicatedRealEngTorq_Out) -> EMS_IndicatedRealEngTorq_Ter/1
  EMS_205/6(EMS_RollingCounter_id205_Out) -> EMS_RollingCounter_id205_Ter/1
  EMS_205/7(EMS_CheckSum_205_Out) -> EMS_CheckSum_205_Ter/1
  EMS_205_GND/1 -> EMS_205/1(input)

== system VCU_CS75_12_16_Test/长安CS75底盘程序，20ms一次/Input/DBC转化的messages（存底）/ReceiveMessages1 ==
  EMS_255 : Subsystem
  EMS_255_GND : Ground
  EMS_AccPedal_Ter : Terminator
  EMS_AccpedelError_Ter : Terminator
  EMS_BrakePedalStatus_Ter : Terminator
  EMS_CheckSum_255_Ter : Terminator
  EMS_EngineSpeedError_Ter : Terminator
  EMS_EngineSpeed_Ter : Terminator
  EMS_RollingCounter_id255_Ter : Terminator
  wires:
  EMS_255/1(EMS_BrakePedalStatus_Out) -> EMS_BrakePedalStatus_Ter/1
  EMS_255/2(EMS_AccpedelError_Out) -> EMS_AccpedelError_Ter/1
  EMS_255/3(EMS_EngineSpeedError_Out) -> EMS_EngineSpeedError_Ter/1
  EMS_255/4(EMS_EngineSpeed_Out) -> EMS_EngineSpeed_Ter/1
  EMS_255/5(EMS_AccPedal_Out) -> EMS_AccPedal_Ter/1
  EMS_255/6(EMS_RollingCounter_id255_Out) -> EMS_RollingCounter_id255_Ter/1
  EMS_255/7(EMS_CheckSum_255_Out) -> EMS_CheckSum_255_Ter/1
  EMS_255_GND/1 -> EMS_255/1(input)

== system VCU_CS75_12_16_Test/长安CS75底盘程序，20ms一次/Input/DBC转化的messages（存底）/ReceiveMessages10 ==
  ESP_287 : Subsystem
  ESP_287_GND : Ground
  ESP_CheckSum_Ter : Terminator
  ESP_HBBActiveStatus_Ter : Terminator
  ESP_HBB_Status_Ter : Terminator
  ESP_HDC_Status_Ter : Terminator
  ESP_HHC_Available_Ter : Terminator
  ESP_LatAcceleration_Ter : Terminator
  ESP_LongAccelValid_Ter : Terminator
  ESP_LongAcceleration_Ter : Terminator
  ESP_RollingCounter_Ter : Terminator
  ESP_TODFastOpenRequest_Ter : Terminator
  ESP_TODTorqueMaxLimit_Ter : Terminator
  ESP_YawRate_Status_Ter : Terminator
  ESP_YawRate_Ter : Terminator
  wires:
  ESP_287_GND/1 -> ESP_287/1(input)
  ESP_287/13(ESP_RollingCounter_Out) -> ESP_RollingCounter_Ter/1
  ESP_287/12(ESP_CheckSum_Out) -> ESP_CheckSum_Ter/1
  ESP_287/11(ESP_YawRate_Status_Out) -> ESP_YawRate_Status_Ter/1
  ESP_287/10(ESP_LongAccelValid_Out) -> ESP_LongAccelValid_Ter/1
  ESP_287/9(ESP_HBBActiveStatus_Out) -> ESP_HBBActiveStatus_Ter/1
  ESP_287/8(ESP_HHC_Available_Out) -> ESP_HHC_Available_Ter/1
  ESP_287/7(ESP_HBB_Status_Out) -> ESP_HBB_Status_Ter/1
  ESP_287/6(ESP_YawRate_Out) -> ESP_YawRate_Ter/1
  ESP_287/5(ESP_LongAcceleration_Out) -> ESP_LongAcceleration_Ter/1
  ESP_287/4(ESP_LatAcceleration_Out) -> ESP_LatAcceleration_Ter/1
  ESP_287/3(ESP_TODFastOpenRequest_Out) -> ESP_TODFastOpenRequest_Ter/1
  ESP_287/2(ESP_HDC_Status_Out) -> ESP_HDC_Status_Ter/1
  ESP_287/1(ESP_TODTorqueMaxLimit_Out) -> ESP_TODTorqueMaxLimit_Ter/1

== system VCU_CS75_12_16_Test/长安CS75底盘程序，20ms一次/Input/DBC转化的messages（存底）/ReceiveMessages11 ==
  HU_AEBOnOffSetting_Ter : Terminator
  HU_AEBSetting_551 : Subsystem
  HU_AEBSetting_551_GND : Ground
  HU_FCWSetting_Ter : Terminator
  HU_LCASetting_Ter : Terminator
  wires:
  HU_AEBSetting_551_GND/1 -> HU_AEBSetting_551/1(input)
  HU_AEBSetting_551/3(HU_FCWSetting_Out) -> HU_FCWSetting_Ter/1
  HU_AEBSetting_551/2(HU_LCASetting_Out) -> HU_LCASetting_Ter/1
  HU_AEBSetting_551/1(HU_AEBOnOffSetting_Out) -> HU_AEBOnOffSetting_Ter/1
